simulink model "prueba1_serie"  (R2022a)
settings: Solver=FixedStepAuto  StartTime=0.0  StopTime=inf  FixedStep=0.01  RelTol=1e-3
libraries: instrumentseriallib x3, slrealtimeutilitieslib x2
settings Model: Creator=Usuario  LastModifiedBy=Usuario
settings DebuggingCC: ParameterPrecisionLossMsg=none

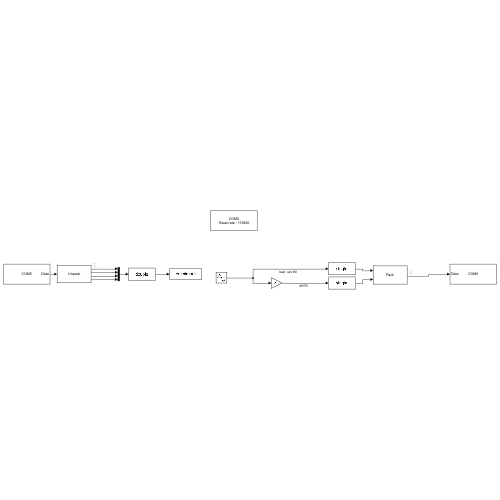
[thumbnail: Simulink's stored preview of the top-level diagram]
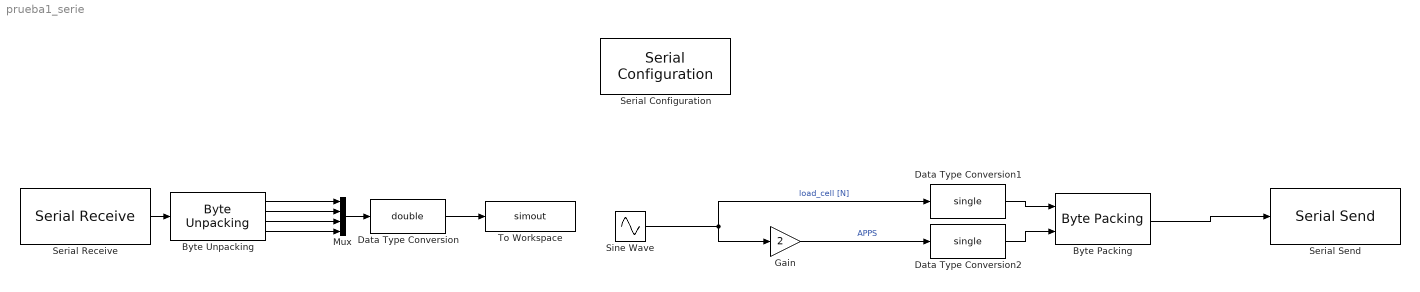
== system prueba1_serie ==
  Byte Packing : slrealtimeutilitieslib/Byte Packing  MaskPackedDataType=uint8  MaskUnpackedDataTypes={'single','single'}  MaskAlignment=1
  Byte Unpacking : slrealtimeutilitieslib/Byte Unpacking  MaskUnpackedDataTypes={'single','single','single','single'}  MaskUnpackedDataSizes={[1],[1],[1],[1]}  MaskAlignment=1
      settings: SourceProductBaseCode=XP
  Data Type Conversion : DataTypeConversion  OutDataTypeStr=double  SaturateOnIntegerOverflow=off  RndMeth=Floor
  Data Type Conversion1 : DataTypeConversion  OutDataTypeStr=single  SaturateOnIntegerOverflow=off  RndMeth=Floor
  Data Type Conversion2 : DataTypeConversion  OutDataTypeStr=single  SaturateOnIntegerOverflow=off  RndMeth=Floor
  Gain : Gain  Gain=2
  Mux : Mux
  Serial Configuration : instrumentseriallib/Serial Configuration  Priority=-200000  PortSel=COM5  Port=COM5  ComPort=COM5  BaudRate=115200  DataBits=8  Parity=none  StopBits=1  ByteOrder=little-endian  FlowControl=none  Timeout=10  SimulateUsing=Interpreted execution  BlockInModel=on  aMode=1
      settings: SourceProductBaseCode=OT,IC,MT
  Serial Receive : instrumentseriallib/Serial Receive  Priority=1  PortSel=COM5  Port=COM5  ComPort=COM5  DataType=uint8  SaveDataType=uint8  ToggleHeader=on  Header=[171 205]  ToggleTerminator=off  Terminator=<none>  CustomTerminator=[]  InputFormat=Column major  ToggleDataSize=on  DataSize=[16 1]  EnableBlockingMode=on  ActionDataUnavailable=Output last received value  ActionWhenDataUnavailable=Output last received value  CustomValue=0  SampleTime=0.01  SimulateUsing=Interpreted execution  BlockInModel=on  aMode=1
      settings: SourceProductBaseCode=OT,IC,MT
  Serial Send : instrumentseriallib/Serial Send  Priority=1  PortSel=COM5  Port=COM5  ComPort=COM5  Header=[202 254]  Terminator=<none>  CustomTerminator=[]  EnableBlockingMode=off  SimulateUsing=Interpreted execution  BlockInModel=on  aMode=1
      settings: SourceProductBaseCode=OT,IC,MT
  Sine Wave : Sin  SineType=Sample based  Bias=1  SampleTime=0.01
  To Workspace : ToWorkspace  VariableName=simout  SampleTime=-1
  wires:
  Data Type Conversion2/1 -> Byte Packing/2
  Data Type Conversion/1 -> To Workspace/1
  Serial Receive/1 -> Byte Unpacking/1
  Byte Unpacking/1 -> Mux/1
  Data Type Conversion1/1 -> Byte Packing/1
  Byte Packing/1 -> Serial Send/1
  Sine Wave/1 -> Data Type Conversion1/1, Gain/1  "load_cell [N]"
  Gain/1 -> Data Type Conversion2/1  "APPS"
  Byte Unpacking/2 -> Mux/2
  Byte Unpacking/3 -> Mux/3
  Byte Unpacking/4 -> Mux/4
  Mux/1 -> Data Type Conversion/1
